simulink model "Detection_Algorithm_Model"  (R2023a)
settings: Solver=VariableStepAuto  StartTime=0.0  StopTime=10.0  RelTol=1e-3
libraries: matrix_library x4, dspsrcs4 x1
settings Model: Creator=Sam Kramer  LastModifiedBy=Sam Kramer

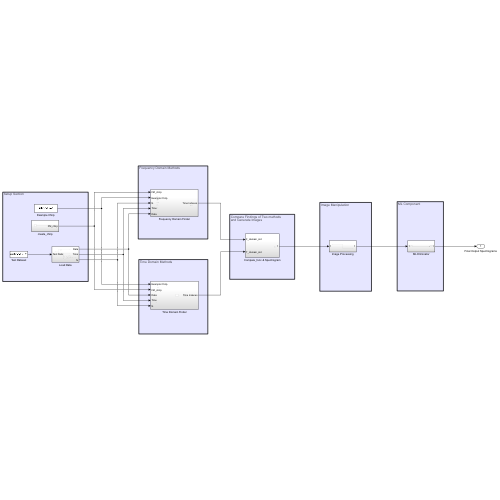
[thumbnail: Simulink's stored preview of the top-level diagram]
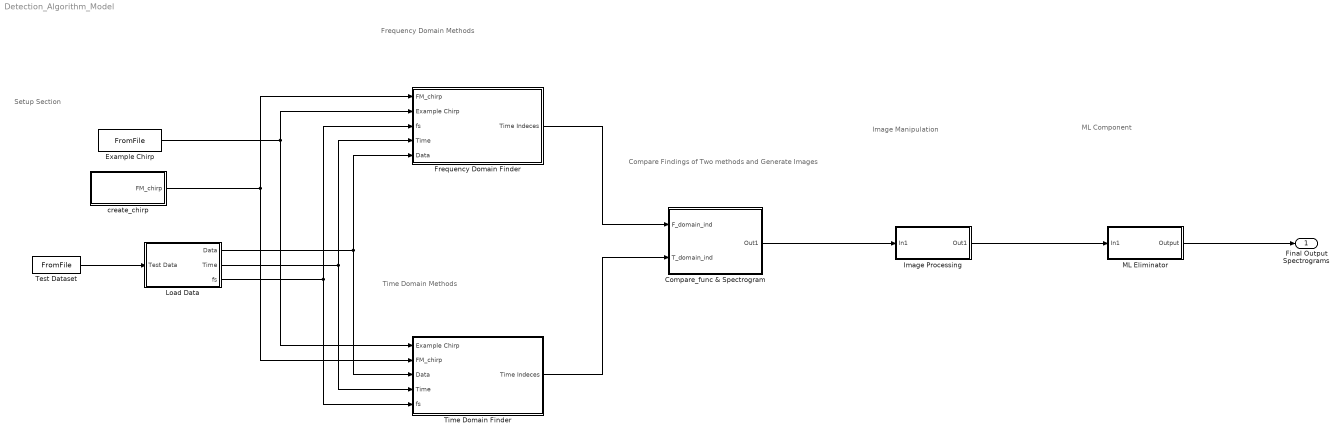
== system Detection_Algorithm_Model ==
  note: Compare Findings of Two methods
      | and Generate Images
  note: ML Component
  note: Image Manipulation
  note: Frequency Domain Methods
  note: Time Domain Methods
  note: Setup Section
  Compare_func & Spectrogram : Subsystem
  Example Chirp : FromFile  SampleTime=0
  Frequency Domain Finder : Subsystem
  Image Processing : Subsystem
  Load Data : Subsystem
  ML Eliminator : Subsystem
  Test Dataset : FromFile  SampleTime=0
  Time Domain Finder : Subsystem
  create_chirp : Subsystem
  Final Output Spectrograms : Outport
  wires:
  Test Dataset/1 -> Load Data/1(Test Data)
  create_chirp/1(FM_chirp) -> Frequency Domain Finder/1(FM_chirp), Time Domain Finder/2(FM_chirp)
  Load Data/1(Data) -> Frequency Domain Finder/5(Data), Time Domain Finder/3(Data)
  Load Data/2(Time) -> Frequency Domain Finder/4(Time), Time Domain Finder/4(Time)
  Load Data/3(fs) -> Frequency Domain Finder/3(fs), Time Domain Finder/5(fs)
  Example Chirp/1 -> Time Domain Finder/1(Example Chirp), Frequency Domain Finder/2(Example Chirp)
  Image Processing/1(Out1) -> ML Eliminator/1(In1)
  Frequency Domain Finder/1(Time Indeces) -> Compare_func & Spectrogram/1(F_domain_ind)
  Time Domain Finder/1(Time Indeces) -> Compare_func & Spectrogram/2(T_domain_ind)
  Compare_func & Spectrogram/1(Out1) -> Image Processing/1(In1)
  ML Eliminator/1(Output) -> Final Output Spectrograms/1

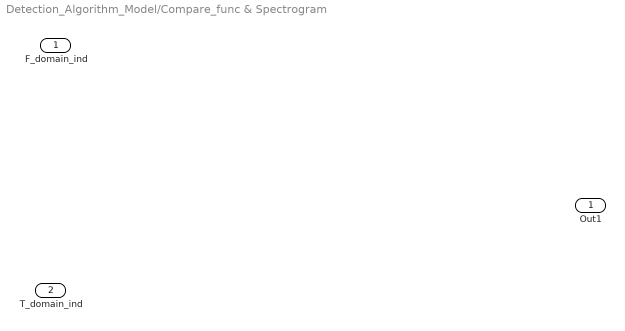
== system Detection_Algorithm_Model/Compare_func & Spectrogram ==
  F_domain_ind : Inport
  T_domain_ind : Inport  Port=2
  Out1 : Outport

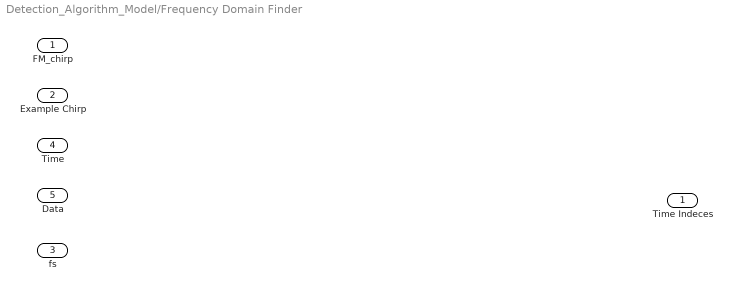
== system Detection_Algorithm_Model/Frequency Domain Finder ==
  FM_chirp : Inport
  Example Chirp : Inport  Port=2
  fs : Inport  Port=3
  Time : Inport  Port=4
  Data : Inport  Port=5
  Time Indeces : Outport

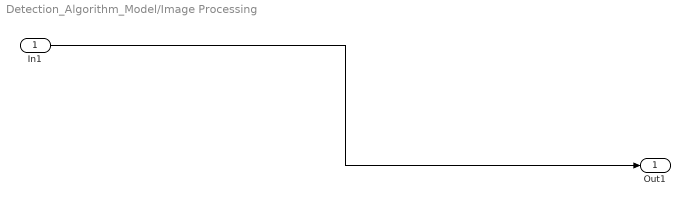
== system Detection_Algorithm_Model/Image Processing ==
  In1 : Inport
  Out1 : Outport
  wires:
  In1/1 -> Out1/1

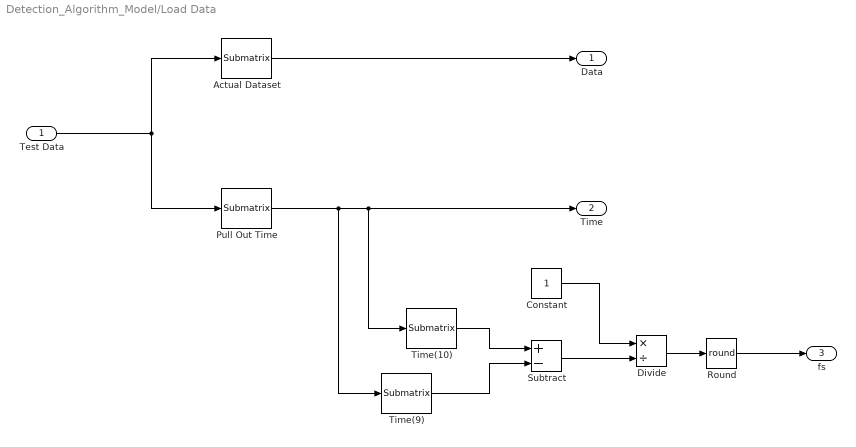
== system Detection_Algorithm_Model/Load Data ==
  Test Data : Inport
  Actual Dataset : matrix_library/Submatrix  RowSpan=All rows  RowStartMode=First  RowStartIndex=1  RowEndMode=Last  RowEndIndex=1  ColSpan=Range of columns  ColStartMode=Index  ColStartIndex=2  ColEndMode=Last  ColEndIndex=1
  Constant : Constant
  Divide : Product  Inputs=*/
  Pull Out Time : matrix_library/Submatrix  RowSpan=All rows  RowStartMode=First  RowStartIndex=1  RowEndMode=Last  RowEndIndex=1  ColSpan=One column  ColStartMode=First  ColStartIndex=1  ColEndMode=Last  ColEndIndex=1
  Round : Rounding  Operator=round
  Subtract : Sum  Inputs=+-
  Time(10) : matrix_library/Submatrix  RowSpan=One row  RowStartMode=Index  RowStartIndex=10  RowEndMode=Last  RowEndIndex=1  ColSpan=All columns  ColStartMode=First  ColStartIndex=1  ColEndMode=Last  ColEndIndex=1
  Time(9) : matrix_library/Submatrix  RowSpan=One row  RowStartMode=Index  RowStartIndex=9  RowEndMode=Last  RowEndIndex=1  ColSpan=All columns  ColStartMode=First  ColStartIndex=1  ColEndMode=Last  ColEndIndex=1
  Data : Outport
  Time : Outport  Port=2
  fs : Outport  Port=3
  wires:
  Test Data/1 -> Actual Dataset/1, Pull Out Time/1
  Actual Dataset/1 -> Data/1
  Pull Out Time/1 -> Time(10)/1, Time/1, Time(9)/1
  Time(9)/1 -> Subtract/2
  Time(10)/1 -> Subtract/1
  Constant/1 -> Divide/1
  Subtract/1 -> Divide/2
  Divide/1 -> Round/1
  Round/1 -> fs/1

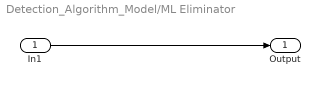
== system Detection_Algorithm_Model/ML Eliminator ==
  In1 : Inport
  Output : Outport
  wires:
  In1/1 -> Output/1

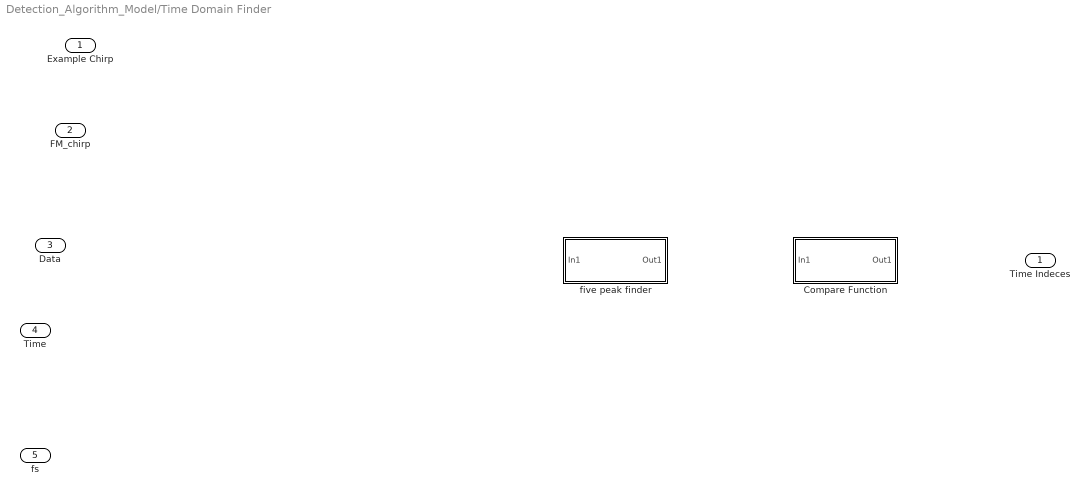
== system Detection_Algorithm_Model/Time Domain Finder ==
  Example Chirp : Inport
  FM_chirp : Inport  Port=2
  Data : Inport  Port=3
  Time : Inport  Port=4
  fs : Inport  Port=5
  Compare Function : Subsystem
  five peak finder : Subsystem
  Time Indeces : Outport

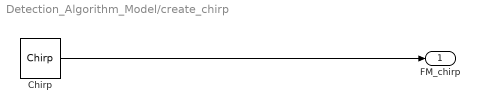
== system Detection_Algorithm_Model/create_chirp ==
  Chirp : dspsrcs4/Chirp  sweep=Linear  mode=Unidirectional  f0=120000  f1=100000  t1=1  Tsweep=1  phase=0  Ts=1/500000  spf=500000*0.005  datatype=Double  OutputFrames=off
  FM_chirp : Outport
  wires:
  Chirp/1 -> FM_chirp/1

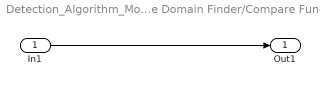
== system Detection_Algorithm_Model/Time Domain Finder/Compare Function ==
  In1 : Inport
  Out1 : Outport
  wires:
  In1/1 -> Out1/1

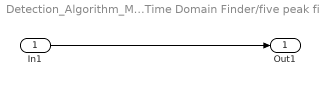
== system Detection_Algorithm_Model/Time Domain Finder/five peak finder ==
  In1 : Inport
  Out1 : Outport
  wires:
  In1/1 -> Out1/1
